simulink model "Deliverable1_Pacemaker"  (R2020a)
settings: Solver=FixedStepAuto  StartTime=0.0  StopTime=1.5  FixedStep=1e-3  RelTol=1e-3  EnableMultiTasking=on
undefined symbols (not defined in the file): D0, D1, D10, D11, D12, D13, D2, D3, D4, D5, D6, D7, D8, D9, PTA0, PTA1, PTA2, PTB23, PTB9, PTC16, PTC17, PTC2, PTC3, PTC4, PTD0, PTD1, PTD2, PTD3
libraries: frdmk64flib x14
settings Model: EnablePacing=on  PacingRate=0.089000  ExtModeTrigDuration=5  Creator=Qingchao  LastModifiedBy=Karolinka
settings OptimizationCC: EnhancedBackFolding=on  PassReuseOutputArgsAs=Individual arguments  ZeroExternalMemoryAtStartup=off  ZeroInternalMemoryAtStartup=off  MaxStackSize=64  OptimizeBlockOrder=speed  DifferentSizesBufferReuse=on  OptimizationCustomize=off  EfficientTunableParamExpr=on
settings DebuggingCC: ParameterTunabilityLossMsg=error
settings HardwareCC: ProdBitPerPointer=32  ProdBitPerSizeT=32  ProdBitPerPtrDiffT=32  ProdLargestAtomicInteger=Long  ProdLargestAtomicFloat=Double  ProdWordSize=32  ProdHWDeviceType=ARM Compatible->ARM Cortex
settings SFSimCC: MATLABDynamicMemAlloc=off
settings RTWCC: SystemTargetFile=ert.tlc  HardwareBoard=NXP FRDM-K64F  TemplateMakefile=ert_default_tmf  Toolchain=GNU Tools for ARM Embedded Processors
settings CodeAppCC: ForceParamTrailComments=on  IgnoreCustomStorageClasses=off  OperatorAnnotations=on  SimulinkDataObjDesc=on  SFDataObjDesc=on  InsertBlockDesc=on

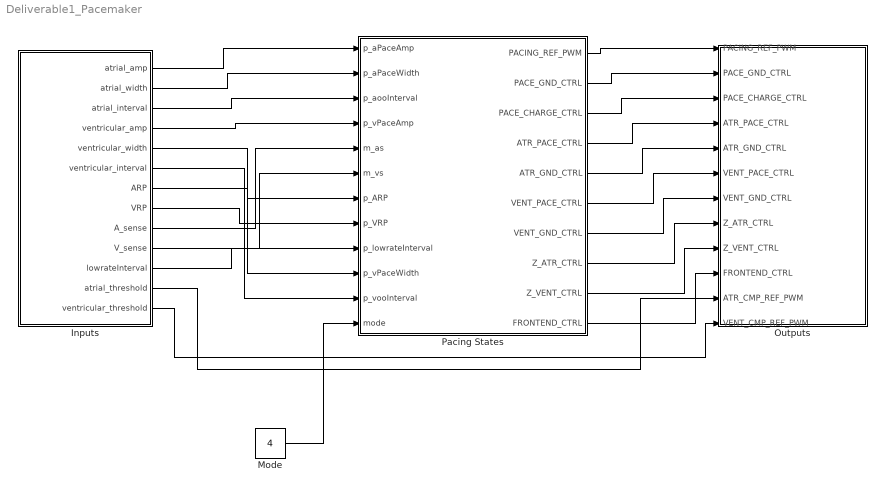
== system Deliverable1_Pacemaker ==
  Inputs : Subsystem
  Mode : Constant  Value=4
  Outputs : Subsystem
  Pacing States : Stateflow chart  TreatAsAtomicUnit=on
      settings: PortSchema="{\"entries\":[{\"content\":{\"sides\":[{\"content\":{\"connectorIds\":[\"In1\",\"In2\",\"In3\",\"In7\",\"In8\",\"In9\",\"In10\",\"In11\",\"In12\",\"In6\",\"In5\",\"In4\"]},\"type\":\"ConnectorPlacement.EquallySpacedRectSide\",\"uuid\":\"0802502d-289b-4258-bc43-1fdd19e28146\"},{\"content\":{\"connectorIds\":[\"Out1\",\"Out2\",\"Out3\",\"Out4\",\"Out5\",\"Out6\",\"Out7\",\"Out8\",\"Out9\",\"Out10\"],\"side\":\"RIGHT\"},\"type\":\"ConnectorPlacement.EquallySpacedRectSide\",\"uuid\":\"3799e012-452c-4265-b73c-d6aca0a0547e\"},{\"content\":{\"connectorIds\":[],\"side\":\"TOP\"},\"type\":\"ConnectorPlacement.EquallySpacedRectSide\",\"uuid\":\"c85fe68a-0875-4c29-a186-d123845da7d6\"}]},\"type\":\"ConnectorPlacement.EquallySpacedConnector\",\"uuid\":\"b828e4d9-145f-473b-83f4-1c85a4420187\"}],\"packageUris\":[\"http://schema.mathworks.com/mf0/Connector/19700101\"],\"version\":\"1.0\"}"
  wires:
  Mode/1 -> Pacing States/4(mode)
  Inputs/1(atrial_amp) -> Pacing States/1(p_aPaceAmp)
  Inputs/2(atrial_width) -> Pacing States/2(p_aPaceWidth)
  Inputs/3(atrial_interval) -> Pacing States/3(p_aooInterval)
  Inputs/5(ventricular_width) -> Pacing States/6(p_vPaceWidth)
  Inputs/4(ventricular_amp) -> Pacing States/7(p_vPaceAmp)
  Inputs/6(ventricular_interval) -> Pacing States/5(p_vooInterval)
  Pacing States/1(PACING_REF_PWM) -> Outputs/1(PACING_REF_PWM)
  Pacing States/2(PACE_GND_CTRL) -> Outputs/2(PACE_GND_CTRL)
  Pacing States/3(PACE_CHARGE_CTRL) -> Outputs/3(PACE_CHARGE_CTRL)
  Pacing States/4(ATR_PACE_CTRL) -> Outputs/4(ATR_PACE_CTRL)
  Pacing States/5(ATR_GND_CTRL) -> Outputs/5(ATR_GND_CTRL)
  Pacing States/6(VENT_PACE_CTRL) -> Outputs/6(VENT_PACE_CTRL)
  Pacing States/7(VENT_GND_CTRL) -> Outputs/7(VENT_GND_CTRL)
  Inputs/7(ARP) -> Pacing States/10(p_ARP)
  Inputs/8(VRP) -> Pacing States/11(p_VRP)
  Inputs/9(A_sense) -> Pacing States/8(m_as)
  Inputs/10(V_sense) -> Pacing States/9(m_vs)
  Inputs/11(lowrateInterval) -> Pacing States/12(p_lowrateInterval)
  Pacing States/8(Z_ATR_CTRL) -> Outputs/8(Z_ATR_CTRL)
  Pacing States/9(Z_VENT_CTRL) -> Outputs/9(Z_VENT_CTRL)
  Pacing States/10(FRONTEND_CTRL) -> Outputs/10(FRONTEND_CTRL)
  Inputs/12(atrial_threshold) -> Outputs/11(ATR_CMP_REF_PWM)
  Inputs/13(ventricular_threshold) -> Outputs/12(VENT_CMP_REF_PWM)

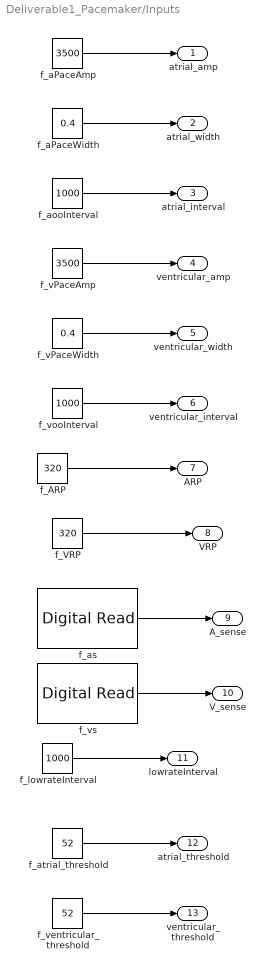
== system Deliverable1_Pacemaker/Inputs ==
  f_ARP : Constant  Value=320
  f_VRP : Constant  Value=320
  f_aPaceAmp : Constant  Value=3500  VectorParams1D=off
  f_aPaceWidth : Constant  Value=0.4
  f_aooInterval : Constant  Value=1000
  f_as : frdmk64flib/Digital Read  Whichpin=PTC16 (D0)  SampleTime=-1
  f_atrial_threshold : Constant  Value=52  VectorParams1D=off
  f_lowrateInterval : Constant  Value=1000
  f_vPaceAmp : Constant  Value=3500  VectorParams1D=off
  f_vPaceWidth : Constant  Value=0.4
  f_ventricular_threshold : Constant  Value=52
  f_vooInterval : Constant  Value=1000
  f_vs : frdmk64flib/Digital Read  Whichpin=PTC17 (D1)  SampleTime=-1
  atrial_amp : Outport
  atrial_width : Outport  Port=2
  atrial_interval : Outport  Port=3
  ventricular_amp : Outport  Port=4
  ventricular_width : Outport  Port=5
  ventricular_interval : Outport  Port=6
  ARP : Outport  Port=7
  VRP : Outport  Port=8
  A_sense : Outport  Port=9
  V_sense : Outport  Port=10
  lowrateInterval : Outport  Port=11
  atrial_threshold : Outport  Port=12
  ventricular_threshold : Outport  Port=13
  wires:
  f_aPaceAmp/1 -> atrial_amp/1
  f_aPaceWidth/1 -> atrial_width/1
  f_aooInterval/1 -> atrial_interval/1
  f_vPaceAmp/1 -> ventricular_amp/1
  f_vPaceWidth/1 -> ventricular_width/1
  f_vooInterval/1 -> ventricular_interval/1
  f_ARP/1 -> ARP/1
  f_VRP/1 -> VRP/1
  f_as/1 -> A_sense/1
  f_vs/1 -> V_sense/1
  f_lowrateInterval/1 -> lowrateInterval/1
  f_atrial_threshold/1 -> atrial_threshold/1
  f_ventricular_threshold/1 -> ventricular_threshold/1

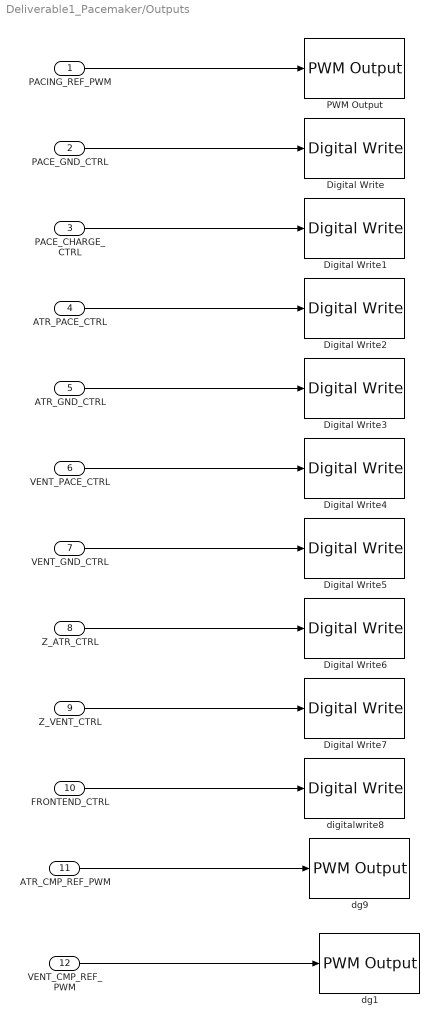
== system Deliverable1_Pacemaker/Outputs ==
  PACING_REF_PWM : Inport
  PACE_GND_CTRL : Inport  Port=2
  PACE_CHARGE_CTRL : Inport  Port=3
  ATR_PACE_CTRL : Inport  Port=4
  ATR_GND_CTRL : Inport  Port=5
  VENT_PACE_CTRL : Inport  Port=6
  VENT_GND_CTRL : Inport  Port=7
  Z_ATR_CTRL : Inport  Port=8
  Z_VENT_CTRL : Inport  Port=9
  FRONTEND_CTRL : Inport  Port=10
  ATR_CMP_REF_PWM : Inport  Port=11
  VENT_CMP_REF_PWM : Inport  Port=12
  Digital Write : frdmk64flib/Digital Write  Whichpin=PTD0 (D10)
  Digital Write1 : frdmk64flib/Digital Write  Whichpin=PTB9 (D2)
  Digital Write2 : frdmk64flib/Digital Write  Whichpin=PTA0 (D8)
  Digital Write3 : frdmk64flib/Digital Write  Whichpin=PTD2 (D11)
  Digital Write4 : frdmk64flib/Digital Write  Whichpin=PTC4 (D9)
  Digital Write5 : frdmk64flib/Digital Write  Whichpin=PTD3 (D12)
  Digital Write6 : frdmk64flib/Digital Write  Whichpin=PTB23 (D4)
  Digital Write7 : frdmk64flib/Digital Write  Whichpin=PTC3 (D7)
  PWM Output : frdmk64flib/PWM Output  Whichpin=PTA2 (D5)  InitialFrequency=2000  InitialDutyCycle=0
  dg1 : frdmk64flib/PWM Output  Whichpin=PTA1 (D3)  InitialFrequency=2000  InitialDutyCycle=70
  dg9 : frdmk64flib/PWM Output  Whichpin=PTC2 (D6)  InitialFrequency=2000  InitialDutyCycle=70
  digitalwrite8 : frdmk64flib/Digital Write  Whichpin=PTD1 (D13)
  wires:
  PACING_REF_PWM/1 -> PWM Output/1
  PACE_GND_CTRL/1 -> Digital Write/1
  PACE_CHARGE_CTRL/1 -> Digital Write1/1
  ATR_PACE_CTRL/1 -> Digital Write2/1
  ATR_GND_CTRL/1 -> Digital Write3/1
  VENT_GND_CTRL/1 -> Digital Write5/1
  VENT_PACE_CTRL/1 -> Digital Write4/1
  Z_ATR_CTRL/1 -> Digital Write6/1
  Z_VENT_CTRL/1 -> Digital Write7/1
  FRONTEND_CTRL/1 -> digitalwrite8/1
  ATR_CMP_REF_PWM/1 -> dg9/1
  VENT_CMP_REF_PWM/1 -> dg1/1

== stateflow chart Deliverable1_Pacemaker/Pacing States ==
  state Initialization
    entry:
    PACE_CHARGE_CTRL = 0
    PACE_GND_CTRL = 0
    ATR_PACE_CTRL = 0
    ATR_GND_CTRL = 0
    VENT_GND_CTRL = 0
    VENT_PACE_CTRL = 0
    PACING_REF_PWM = 0
  state AOO
    entry:
    FRONTEND_CTRL = 0;
    state Discharging_C21
      entry:
      PACE_GND_CTRL = 1
      ATR_PACE_CTRL = 0
      %Z_ATR_CTRL = 0
      %Z_VENT_CTRL = 0
      %VENT_PACE_CTRL = 0
      %VENT_GND_CTRL = 0
      ATR_GND_CTRL = 1
    state Pacing_atrium
      entry:
      PACE_CHARGE_CTRL = 0
      PACE_GND_CTRL = 1
      ATR_PACE_CTRL = 1
      ATR_GND_CTRL = 0
      %Z_ATR_CTRL = 0
      %Z_VENT_CTRL = 0
      %VENT_GND_CTRL = 0
      %VENT_PACE_CTRL = 0
      PACING_REF_PWM = 0
    state Charging_C22
      entry:
      ATR_PACE_CTRL = 0
      %VENT_PACE_CTRL = 0
      PACING_REF_PWM = p_aPaceAmp/max_V*100
      PACE_CHARGE_CTRL = 1
    (default) -> AOO.Discharging_C21
    AOO.Pacing_atrium -> AOO.Discharging_C21 : after(p_aPaceWidth, msec)
    AOO.Discharging_C21 -> AOO.Charging_C22
    AOO.Charging_C22 -> AOO.Pacing_atrium : [after(p_aooInterval-p_aPaceWidth, msec) ]
  state VOO
    entry:
    FRONTEND_CTRL = 0;
    state Discharging_C21
      entry:
      PACE_GND_CTRL = 1
      %ATR_PACE_CTRL = 0
      %Z_ATR_CTRL = 0
      %Z_VENT_CTRL = 0
      VENT_PACE_CTRL = 0
      VENT_GND_CTRL = 1
      %ATR_GND_CTRL = 1
    state Pacing_ventricle
      entry:
      PACE_CHARGE_CTRL = 0
      PACE_GND_CTRL = 1
      %ATR_PACE_CTRL = 1
      %ATR_GND_CTRL = 0
      %Z_ATR_CTRL = 0
      %Z_VENT_CTRL = 0
      VENT_PACE_CTRL = 1
      VENT_GND_CTRL = 0
      PACING_REF_PWM = 0
    state Charging_C22
      entry:
      %ATR_PACE_CTRL = 0
      VENT_PACE_CTRL = 0
      PACING_REF_PWM = p_vPaceAmp/max_V*100
      PACE_CHARGE_CTRL = 1
    (default) -> VOO.Discharging_C21
    VOO.Pacing_ventricle -> VOO.Discharging_C21 : after(p_vPaceWidth, msec)
    VOO.Discharging_C21 -> VOO.Charging_C22
    VOO.Charging_C22 -> VOO.Pacing_ventricle : [after(p_vooInterval-p_vPaceWidth, msec) ]
  state AAI
    entry:
    FRONTEND_CTRL = 1;
    state Discharging_C21
      entry:
      PACE_GND_CTRL = 1
      VENT_PACE_CTRL = 0
      Z_ATR_CTRL = 0
      Z_VENT_CTRL = 0
      ATR_PACE_CTRL = 0
      ATR_GND_CTRL = 1
      VENT_GND_CTRL = 0
    state Pacing_atrium
      entry:
      PACE_CHARGE_CTRL = 0
      PACE_GND_CTRL = 1
      ATR_PACE_CTRL = 1
      ATR_GND_CTRL = 0
      Z_ATR_CTRL = 0
      Z_VENT_CTRL = 0
      VENT_GND_CTRL = 0
      VENT_PACE_CTRL = 0
    state ARP
    state Charging_C22
      entry:
      ATR_PACE_CTRL = 0
      VENT_PACE_CTRL = 0
      PACING_REF_PWM = p_aPaceAmp/max_V*100
      PACE_CHARGE_CTRL = 1
    (default) -> AAI.Discharging_C21
    AAI.Pacing_atrium -> AAI.Discharging_C21 : after(p_aPaceWidth, msec)
    AAI.Discharging_C21 -> ARP
    (junction 145) -> AAI.Pacing_atrium [order 2] : [m_as == 0]
    (junction 145) -> ARP [order 1] : [m_as == 1]
    AAI.Charging_C22 -> (junction 145) [order 1] : [after(p_lowrateInterval-p_aPaceWidth-p_ARP, msec) ]
    AAI.Charging_C22 -> ARP [order 2] : [m_as == 1]
    ARP -> AAI.Charging_C22 : [after(p_ARP,msec)]
  state VVI
    entry:
    FRONTEND_CTRL = 1;
    state Discharging_C21
      entry:
      PACE_GND_CTRL = 1
      VENT_PACE_CTRL = 0
      Z_ATR_CTRL = 0
      Z_VENT_CTRL = 0
      ATR_PACE_CTRL = 0
      ATR_GND_CTRL = 0
      VENT_GND_CTRL = 1
    state Pacing_ventricle
      entry:
      PACE_CHARGE_CTRL = 0
      PACE_GND_CTRL = 1
      ATR_PACE_CTRL = 0
      ATR_GND_CTRL = 0
      Z_ATR_CTRL = 0
      Z_VENT_CTRL = 0
      VENT_GND_CTRL = 0
      VENT_PACE_CTRL = 1
    state VRP
    state Charging_C22
      entry:
      ATR_PACE_CTRL = 0
      VENT_PACE_CTRL = 0
      PACING_REF_PWM = p_vPaceAmp/max_V*100
      PACE_CHARGE_CTRL = 1
    (default) -> VVI.Discharging_C21
    VVI.Pacing_ventricle -> VVI.Discharging_C21 : after(p_vPaceWidth, msec)
    VVI.Discharging_C21 -> VRP
    (junction 160) -> VVI.Pacing_ventricle [order 2] : [m_vs == 0]
    (junction 160) -> VRP [order 1] : [m_vs == 1]
    VVI.Charging_C22 -> (junction 160) [order 1] : [after(p_lowrateInterval-p_vPaceWidth-p_VRP, msec) ]
    VVI.Charging_C22 -> VRP [order 2] : [m_vs == 1]
    VRP -> VVI.Charging_C22 : [after(p_VRP,msec)]
  (default) -> Initialization
  Initialization -> VVI [order 4] : [mode == 4]
  Initialization -> AOO [order 1] : [mode == 1]
  Initialization -> VOO [order 2] : [mode == 2]
  Initialization -> AAI [order 3] : [mode == 3]
  data: p_aPaceAmp input; p_aPaceWidth input; p_aooInterval input; max_V constant double =5000; PACING_REF_PWM output; PACE_GND_CTRL output; PACE_CHARGE_CTRL output; ATR_PACE_CTRL output; ATR_GND_CTRL output; VENT_PACE_CTRL output; VENT_GND_CTRL output; mode input; p_vooInterval input; p_vPaceWidth input; p_vPaceAmp input; m_as input; m_vs input; p_ARP input; p_VRP input; p_lowrateInterval input; Z_ATR_CTRL output; Z_VENT_CTRL output; FRONTEND_CTRL output
